simulink model "CompletoyLPV"  (R2025a)
settings: Solver=VariableStepAuto  StartTime=0.0  StopTime=10.0  RelTol=1e-3
PostLoadFcn:
  | parametros_sistema_completo
  | run("parametros_sistema_completo.mlx")
values from neighbouring files (symbols this model uses):
  a_cu = 3.9e-3    (= 0.0039)    [parametros_sistema_completo.m]    (also in workspace_params.mat)
  b_eq = params.b_total    [calcular_matriz_AO.m]    (also in calculo_incertidumbre_y_control.m = b_m + b_l/(r^2); parametros_sistema_completo.m = 2.19444444444e-05; workspace_params.mat = 2.19444444444e-05)
  C_ts = C_ts * (1 + tol_pct)    [calculo_incertidumbre_y_control.m]    (also in parametros_sistema_completo.m = 0.818; workspace_params.mat = 0.818)
  g = 9.80665    [parametros_sistema_completo.m]    (also in workspace_params.mat)
  J_eq = params.J_total    [calcular_matriz_AO.m]    (also in calculo_incertidumbre_y_control.m = J_m + J_l/r^2; parametros_sistema_completo.m = 1.97847222222e-05; workspace_params.mat = 3.28055555556e-05)
  k_l = m*l_cm + m_l*l_l    [calculo_incertidumbre_y_control.m]    (also in parametros_sistema_completo.m = 0.25; workspace_params.mat = 0.625)
  L_d = L_d    * (1 - tol_pct)    [calculo_incertidumbre_y_control.m]    (also in parametros_sistema_completo.m = 0.0066; workspace_params.mat = 0.0066)
  L_ls = L_ls   * (1 - tol_pct)    [calculo_incertidumbre_y_control.m]    (also in parametros_sistema_completo.m = 0.0008; workspace_params.mat = 0.0008)
  L_q = L_q    * (1 - tol_pct)    [calculo_incertidumbre_y_control.m]    (also in parametros_sistema_completo.m = 0.0058; workspace_params.mat = 0.0058)
  lambda_r = lambda_r * (1 + tol_pct)    [calculo_incertidumbre_y_control.m]    (also in parametros_sistema_completo.m = 0.016; workspace_params.mat = 0.016)
  P_p = 3    [parametros_sistema_completo.m]    (also in workspace_params.mat)
  r = params.r_red    [calcular_matriz_AO.m]    (also in parametros_sistema_completo.m = 120; workspace_params.mat = 120)
  R_sREF = R_sREF * (1 - tol_pct)    [calculo_incertidumbre_y_control.m]    (also in parametros_sistema_completo.m = 1.02; workspace_params.mat = 1.02)
  R_ts_amb = R_ts_amb * (1 - tol_pct)    [calculo_incertidumbre_y_control.m]    (also in parametros_sistema_completo.m = 146.7; workspace_params.mat = 146.7)
  s = max(diff(xl),diff(yl)); xlim(mean(xl)+[-1 1]*s/2); ylim(mean(yl)+[-1 1]*s/2); axis square    [mapa_polos_5_2_2.m]    (also in metricas_5_1_6b.m = iqs(idx); modulador_torque_521.m = tf('s'))
  T_amb = 20    [parametros_sistema_completo.m]    (also in workspace_params.mat)
  T_sREF = 20    [parametros_sistema_completo.m]    (also in workspace_params.mat)
undefined symbols (not defined in the file or in its folder): deg, rad
libraries: aerolibconvert2 x1
settings Model: Creator=Francisco  LastModifiedBy=Francisco
settings DebuggingCC: UnderspecifiedInitializationDetection=Classic  MergeDetectMultiDrivingBlocksExec=none
settings ModelReferenceCC: PropagateSignalLabelsOutOfModel=off
settings RTWCC: GPUComputeCapability=3.5

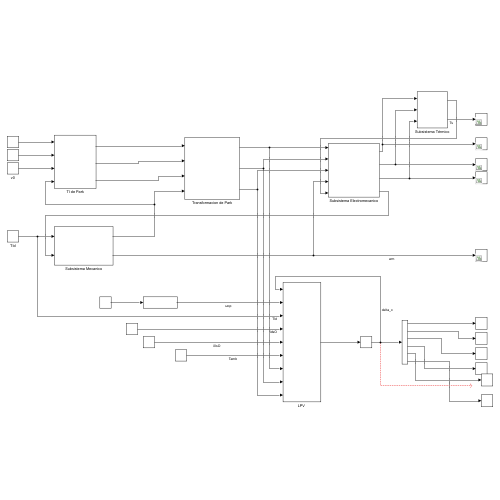
[thumbnail: Simulink's stored preview of the top-level diagram]
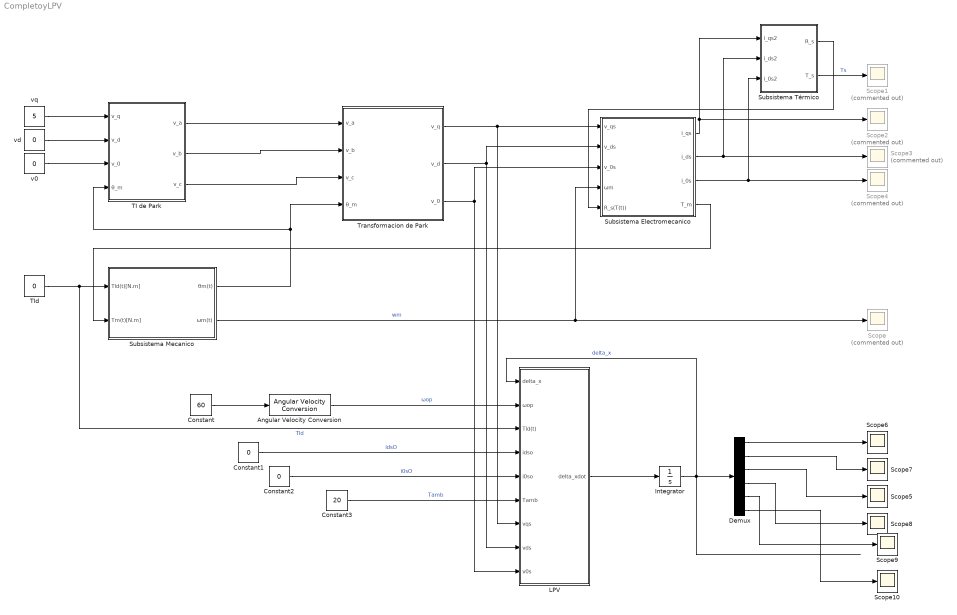
== system CompletoyLPV ==
  Angular Velocity Conversion : aerolibconvert2/Angular Velocity Conversion  IU=deg/s  OU=rad/s
  Constant : Constant  Value=60
  Constant1 : Constant  Value=0
  Constant2 : Constant  Value=0
  Constant3 : Constant  Value=20
  Demux : Demux  Outputs=6
  Integrator : Integrator
  "LPV " : Subsystem
  Scope{,1..4} (5 alike) : Scope  Commented=on
      Scope settings: ActiveDisplayYMinimum=73.83566  ActiveDisplayYMaximum=91.14361
      Scope1 settings: ActiveDisplayYMinimum=-0.21459  ActiveDisplayYMaximum=1.93128
      Scope2 settings: ActiveDisplayYMinimum=-0.79232  ActiveDisplayYMaximum=3.09165  DataLoggingVariableName=ScopeData2
      Scope3 settings: ActiveDisplayYMinimum=-0.21509  ActiveDisplayYMaximum=1.75287  DataLoggingVariableName=ScopeData3
      Scope4 settings: ActiveDisplayYMinimum=-4.8E-11  ActiveDisplayYMaximum=5E-11  DataLoggingVariableName=ScopeData4
  Scope{5..10} (6 alike) : Scope
      Scope10 settings: ActiveDisplayYMinimum=1.2614013021411665  ActiveDisplayYMaximum=31.468208023043097  DataLoggingVariableName=ScopeData10
      Scope5 settings: ActiveDisplayYMinimum=-67.200227328003422  ActiveDisplayYMaximum=44.635452648293487  DataLoggingVariableName=ScopeData5
      Scope6 settings: ActiveDisplayYMinimum=-60.0071453689453  ActiveDisplayYMaximum=12.244259941879115  DataLoggingVariableName=ScopeData6
      Scope7 settings: ActiveDisplayYMinimum=-3.8566133388452828  ActiveDisplayYMaximum=11.094644624657567  DataLoggingVariableName=ScopeData7
      Scope8 settings: ActiveDisplayYMinimum=-4.8085485964497172  ActiveDisplayYMaximum=10.142709367053149  DataLoggingVariableName=ScopeData8
      Scope9 settings: ActiveDisplayYMinimum=-7.1222346828694452  ActiveDisplayYMaximum=12.913880935880563  DataLoggingVariableName=ScopeData9
  Subsistema Electromecanico : Subsystem
  Subsistema Mecanico : Subsystem
  Subsistema Térmico : Subsystem
  TI de Park : Subsystem
  TId : Constant  Value=0
  Transformacion de Park : Subsystem
  v0 : Constant  Value=0
  vd : Constant  Value=0
  vq : Constant  Value=5
  wires:
  Transformacion de Park/3(v_0) -> Subsistema Electromecanico/3(v_0s), "LPV "/9(v0s)
  Transformacion de Park/2(v_d) -> Subsistema Electromecanico/2(v_ds), "LPV "/8(vds)
  Transformacion de Park/1(v_q) -> "LPV "/7(vqs), Subsistema Electromecanico/1(v_qs)
  Subsistema Térmico/1(R_s) -> Subsistema Electromecanico/5(R_s(T(t)))
  Subsistema Electromecanico/2(i_ds) -> Subsistema Térmico/2(i_ds2), Scope3/1
  Subsistema Térmico/2(T_s) -> Scope1/1  "Ts"
  vq/1 -> TI de Park/1(v_q)
  vd/1 -> TI de Park/2(v_d)
  v0/1 -> TI de Park/3(v_0)
  Subsistema Mecanico/1(θm(t)) -> Transformacion de Park/4(θ_m), TI de Park/4(θ_m)
  Subsistema Mecanico/2(ωm(t)) -> Scope/1, Subsistema Electromecanico/4(ωm)  "wm"
  TI de Park/3(v_c) -> Transformacion de Park/3(v_c)
  Subsistema Electromecanico/1(i_qs) -> Scope2/1, Subsistema Térmico/1(i_qs2)
  Subsistema Electromecanico/3(i_0s) -> Scope4/1, Subsistema Térmico/3(i_0s2)
  Subsistema Electromecanico/4(T_m) -> Subsistema Mecanico/2(Tm(t)[N.m])
  TI de Park/1(v_a) -> Transformacion de Park/1(v_a)
  TI de Park/2(v_b) -> Transformacion de Park/2(v_b)
  Angular Velocity Conversion/1 -> "LPV "/2(ωop)  "ωop"
  TId/1 -> "LPV "/3(Tld(t)), Subsistema Mecanico/1(Tld(t)[N.m])  "Tld"
  Constant1/1 -> "LPV "/4(idso)  "idsO"
  Constant2/1 -> "LPV "/5(i0so)  "i0sO"
  Constant3/1 -> "LPV "/6(Tamb)  "Tamb"
  "LPV "/1(delta_xdot) -> Integrator/1
  Integrator/1 -> "LPV "/1(delta_x), Demux/1  "delta_x"
  Constant/1 -> Angular Velocity Conversion/1
  Demux/3 -> Scope5/1
  Demux/1 -> Scope6/1
  Demux/2 -> Scope7/1
  Demux/4 -> Scope8/1
  Demux/5 -> Scope9/1
  Demux/6 -> Scope10/1

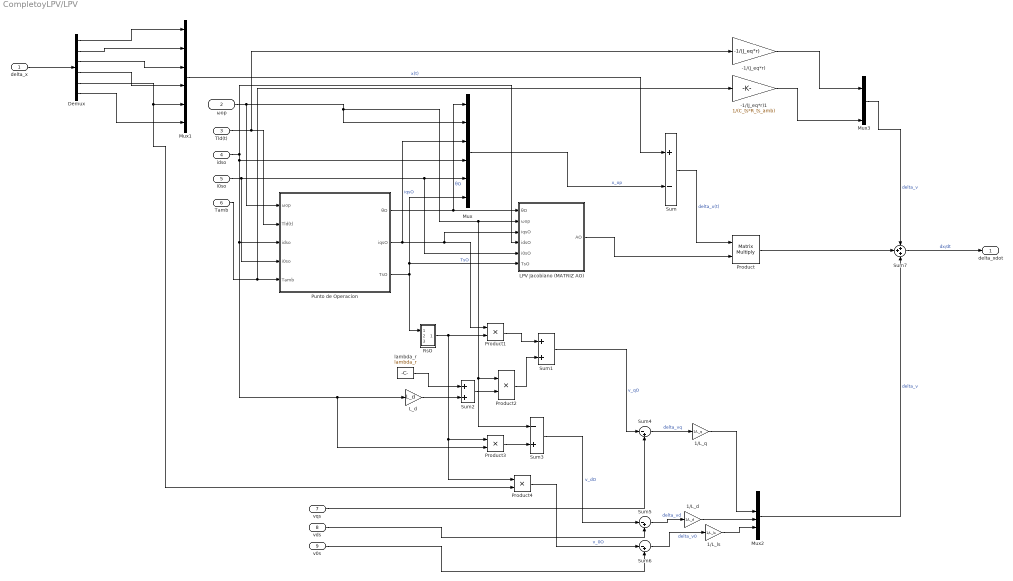
== system CompletoyLPV/LPV  ==
  delta_x : Inport
  ωop : Inport  Port=2
  Tld(t) : Inport  Port=3
  idso : Inport  Port=4
  i0so : Inport  Port=5
  Tamb : Inport  Port=6
  vqs : Inport  Port=7
  vds : Inport  Port=8
  v0s : Inport  Port=9
  -1/(J_eq*r) : Gain  Gain=-1/(J_eq*r)
  -1/(J_eq*r)1 : Gain  Gain=1/(C_ts*R_ts_amb)
  1/L_d : Gain  Gain=1/L_d
  1/L_ls : Gain  Gain=1/L_ls
  1/L_q : Gain  Gain=1/L_q
  Demux : Demux  Outputs=6
  LPV Jacobiano (MATRIZ AO) : Subsystem
  L_d : Gain  Gain=L_d
  Mux{,1..3} (4 alike) : Mux  Inputs=6
  Product : Product  Multiplication=Matrix(*)
  Product{1..4} (4 alike) : Product
  Punto de Operacion : Subsystem
  RsO : MATLAB Function  TreatAsAtomicUnit=on
  Sum : Sum  Inputs=+-
  Sum1 : Sum
  Sum2 : Sum
  Sum3 : Sum  Inputs=-+
  Sum4 : Sum  Inputs=|-+
  Sum5 : Sum  Inputs=|-+
  Sum6 : Sum  Inputs=|-+
  Sum7 : Sum  Inputs=+++
  lambda_r : Constant  Value=lambda_r
  delta_xdot : Outport
  wires:
  Punto de Operacion/2(iqsO) -> Product1/1, LPV Jacobiano (MATRIZ AO)/3(iqsO), Mux/3  "iqsO"
  Mux1/1 -> Sum/1  "x(t)"
  ωop/1 -> Punto de Operacion/1(ωop), LPV Jacobiano (MATRIZ AO)/2(ωop), Sum3/1, Product2/1, Mux/2
  Punto de Operacion/1(θO) -> LPV Jacobiano (MATRIZ AO)/1(θO), Mux/1  "θO"
  Tamb/1 -> -1/(J_eq*r)1/1, Punto de Operacion/5(Tamb)
  i0so/1 -> Mux/5, LPV Jacobiano (MATRIZ AO)/5(i0sO), Punto de Operacion/4(i0so)
  Product/1 -> Sum7/2
  idso/1 -> Mux/4, Punto de Operacion/3(idso), Product3/2, L_d/1, LPV Jacobiano (MATRIZ AO)/4(idsO)
  Mux/1 -> Sum/2  "x_op"
  LPV Jacobiano (MATRIZ AO)/1(AO) -> Product/2
  Sum/1 -> Product/1  "delta_x(t)"
  Tld(t)/1 -> -1/(J_eq*r)/1, Punto de Operacion/2(Tld(t))
  Punto de Operacion/3(TsO) -> RsO/1(TsO), LPV Jacobiano (MATRIZ AO)/6(TsO), Mux/6  "TsO"
  Demux/2 -> Mux1/2
  Demux/6 -> Mux1/6
  Demux/1 -> Mux1/1
  Demux/5 -> Product4/2, Mux1/5
  Demux/4 -> Mux1/4
  Demux/3 -> Mux1/3
  RsO/1(RsO) -> Product4/1, Product3/1, Product1/2
  Product1/1 -> Sum1/1
  L_d/1 -> Sum2/2
  lambda_r/1 -> Sum2/1
  Sum2/1 -> Product2/2
  Product2/1 -> Sum1/2
  Sum1/1 -> Sum4/1  "v_qO"
  Product3/1 -> Sum3/2
  Sum3/1 -> Sum5/1  "v_dO"
  Product4/1 -> Sum6/1  "v_0O"
  vqs/1 -> Sum4/2
  vds/1 -> Sum5/2
  v0s/1 -> Sum6/2
  Mux2/1 -> Sum7/3  "delta_v"
  Sum4/1 -> 1/L_q/1  "delta_vq"
  Sum5/1 -> 1/L_d/1  "delta_vd"
  Sum6/1 -> 1/L_ls/1  "delta_v0"
  1/L_ls/1 -> Mux2/5
  1/L_d/1 -> Mux2/4
  1/L_q/1 -> Mux2/3
  -1/(J_eq*r)/1 -> Mux3/2
  -1/(J_eq*r)1/1 -> Mux3/6
  Mux3/1 -> Sum7/1  "delta_v"
  Sum7/1 -> delta_xdot/1  "dx/dt"
  delta_x/1 -> Demux/1

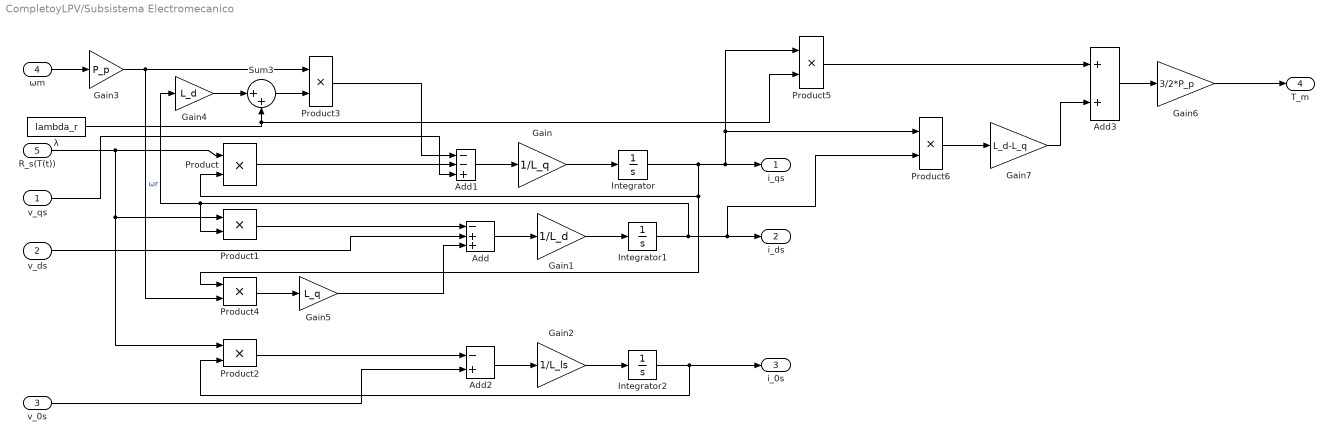
== system CompletoyLPV/Subsistema Electromecanico ==
  v_qs : Inport
  v_ds : Inport  Port=2
  v_0s : Inport  Port=3
  ωm : Inport  Port=4
  R_s(T(t)) : Inport  Port=5
  Add : Sum  Inputs=-++
  Add1 : Sum  Inputs=--+
  Add2 : Sum  Inputs=-+
  Add3 : Sum
  Gain : Gain  Gain=1/L_q
  Gain1 : Gain  Gain=1/L_d
  Gain2 : Gain  Gain=1/L_ls
  Gain3 : Gain  Gain=P_p
  Gain4 : Gain  Gain=L_d
  Gain5 : Gain  Gain=L_q
  Gain6 : Gain  Gain=3/2*P_p
  Gain7 : Gain  Gain=L_d-L_q
  Integrator : Integrator
  Integrator1 : Integrator
  Integrator2 : Integrator
  Product{,1..6} (7 alike) : Product
  Sum3 : Sum  Inputs=|++
  λ : Constant  Value=lambda_r
  i_qs : Outport
  i_ds : Outport  Port=2
  i_0s : Outport  Port=3
  T_m : Outport  Port=4
  wires:
  v_0s/1 -> Add2/2
  Gain5/1 -> Add/3
  Gain3/1 -> Product4/2, Product3/1  "ωr"
  Integrator/1 -> Product4/1, Product/2, i_qs/1, Product5/1, Product6/1
  v_qs/1 -> Add1/3
  R_s(T(t))/1 -> Product2/1, Product1/1, Product/1
  Gain4/1 -> Sum3/1
  Product1/1 -> Add/1
  Integrator2/1 -> i_0s/1, Product2/2
  Sum3/1 -> Product3/2
  Integrator1/1 -> Gain4/1, Product1/2, i_ds/1, Product6/2
  Product/1 -> Add1/2
  Product4/1 -> Gain5/1
  ωm/1 -> Gain3/1
  Add3/1 -> Gain6/1
  Gain/1 -> Integrator/1
  Gain6/1 -> T_m/1
  Product2/1 -> Add2/1
  λ/1 -> Sum3/2, Product5/2
  Gain1/1 -> Integrator1/1
  Add/1 -> Gain1/1
  Add1/1 -> Gain/1
  Product6/1 -> Gain7/1
  Product3/1 -> Add1/1
  Gain2/1 -> Integrator2/1
  Gain7/1 -> Add3/2
  v_ds/1 -> Add/2
  Add2/1 -> Gain2/1
  Product5/1 -> Add3/1

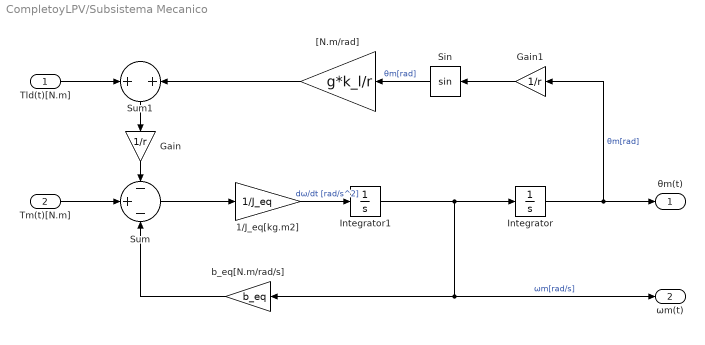
== system CompletoyLPV/Subsistema Mecanico ==
  Tld(t)[N.m] : Inport
  Tm(t)[N.m] : Inport  Port=2
  1/J_eq[kg.m2] : Gain  Gain=1/J_eq
  Gain : Gain  Gain=1/r
  Gain1 : Gain  Gain=1/r
  Integrator : Integrator
  Integrator1 : Integrator
  Sin : Trigonometry
  Sum : Sum  Inputs=-+-
  Sum1 : Sum
  "[N.m/rad]" : Gain  Gain=g*k_l/r
  b_eq[N.m/rad/s] : Gain  Gain=b_eq
  θm(t) : Outport
  ωm(t) : Outport  Port=2
  wires:
  Gain1/1 -> Sin/1
  Sin/1 -> "[N.m/rad]"/1  "θm[rad]"
  Integrator1/1 -> Integrator/1, ωm(t)/1, b_eq[N.m/rad/s]/1  "ωm[rad/s]"
  Tld(t)[N.m]/1 -> Sum1/1
  b_eq[N.m/rad/s]/1 -> Sum/3
  1/J_eq[kg.m2]/1 -> Integrator1/1  "dω/dt [rad/s^2]"
  Gain/1 -> Sum/1
  "[N.m/rad]"/1 -> Sum1/2
  Integrator/1 -> θm(t)/1, Gain1/1  "θm[rad]"
  Sum/1 -> 1/J_eq[kg.m2]/1
  Tm(t)[N.m]/1 -> Sum/2
  Sum1/1 -> Gain/1

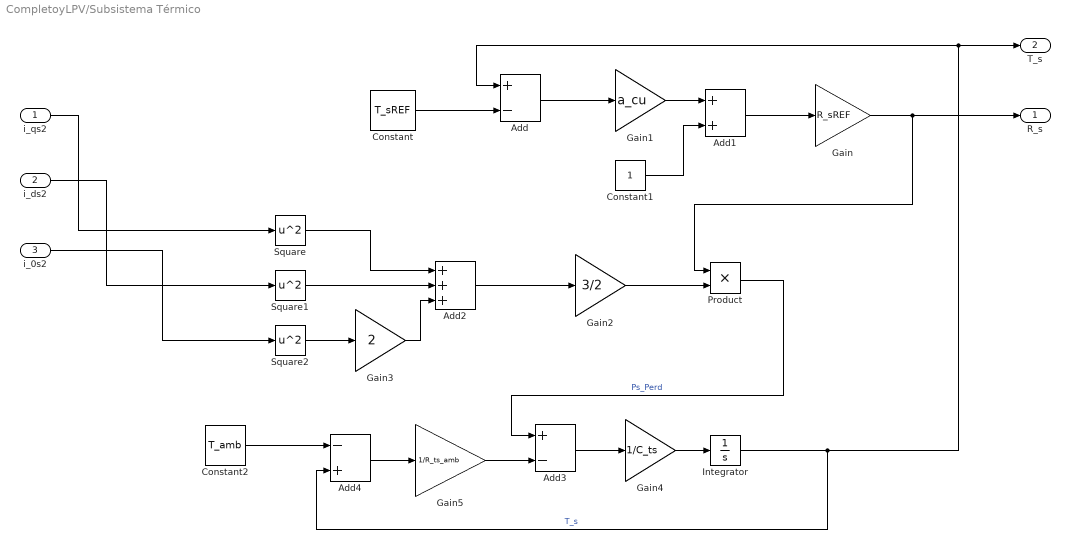
== system CompletoyLPV/Subsistema Térmico ==
  i_qs2 : Inport
  i_ds2 : Inport  Port=2
  i_0s2 : Inport  Port=3
  Add : Sum  Inputs=+-
  Add1 : Sum
  Add2 : Sum  Inputs=+++
  Add3 : Sum  Inputs=+-
  Add4 : Sum  Inputs=-+
  Constant : Constant  Value=T_sREF
  Constant1 : Constant
  Constant2 : Constant  Value=T_amb
  Gain : Gain  Gain=R_sREF
  Gain1 : Gain  Gain=a_cu
  Gain2 : Gain  Gain=3/2
  Gain3 : Gain  Gain=2
  Gain4 : Gain  Gain=1/C_ts
  Gain5 : Gain  Gain=1/R_ts_amb
  Integrator : Integrator
  Product : Product
  Square : Math  Operator=square  OutDataTypeStr=double
  Square1 : Math  Operator=square
  Square2 : Math  Operator=square
  R_s : Outport
  T_s : Outport  Port=2
  wires:
  Constant1/1 -> Add1/2
  Constant/1 -> Add/2
  i_qs2/1 -> Square/1
  Gain/1 -> R_s/1, Product/1
  Square/1 -> Add2/1
  Add2/1 -> Gain2/1
  Constant2/1 -> Add4/1
  i_ds2/1 -> Square1/1
  Gain5/1 -> Add3/2
  Integrator/1 -> Add4/2, T_s/1, Add/1  "T_s"
  Add1/1 -> Gain/1
  i_0s2/1 -> Square2/1
  Square1/1 -> Add2/2
  Product/1 -> Add3/1  "Ps_Perd"
  Gain2/1 -> Product/2
  Add/1 -> Gain1/1
  Square2/1 -> Gain3/1
  Gain1/1 -> Add1/1
  Add3/1 -> Gain4/1
  Add4/1 -> Gain5/1
  Gain3/1 -> Add2/3
  Gain4/1 -> Integrator/1

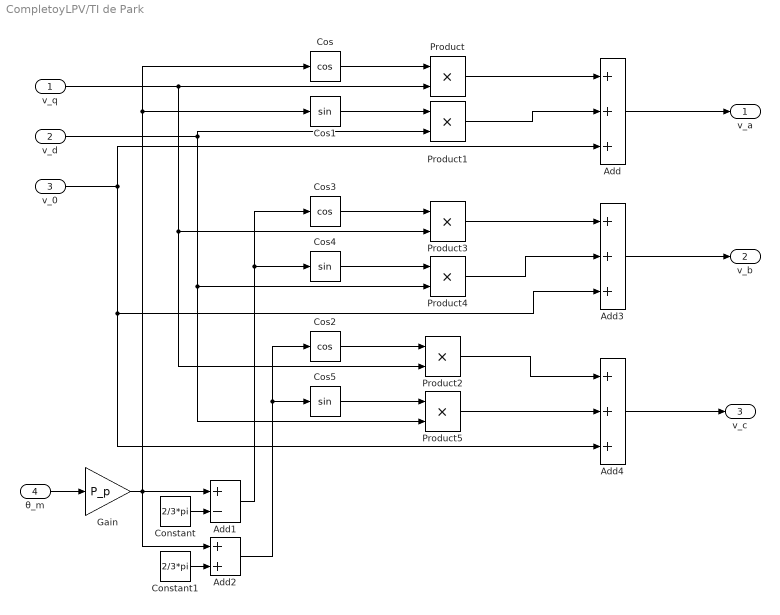
== system CompletoyLPV/TI de Park ==
  v_q : Inport
  v_d : Inport  Port=2
  v_0 : Inport  Port=3
  θ_m : Inport  Port=4
  Add : Sum  Inputs=+++
  Add1 : Sum  Inputs=+-
  Add2 : Sum
  Add3 : Sum  Inputs=+++
  Add4 : Sum  Inputs=+++
  Constant : Constant  Value=2/3*pi
  Constant1 : Constant  Value=2/3*pi
  Cos : Trigonometry  Operator=cos
  Cos1 : Trigonometry
  Cos2 : Trigonometry  Operator=cos
  Cos3 : Trigonometry  Operator=cos
  Cos4 : Trigonometry
  Cos5 : Trigonometry
  Gain : Gain  Gain=P_p
  Product{,1..5} (6 alike) : Product
  v_a : Outport
  v_b : Outport  Port=2
  v_c : Outport  Port=3
  wires:
  Product4/1 -> Add3/2
  Cos1/1 -> Product1/1
  Cos/1 -> Product/1
  Product1/1 -> Add/2
  Add3/1 -> v_b/1
  Cos3/1 -> Product3/1
  Product3/1 -> Add3/1
  v_d/1 -> Product1/2, Product5/2, Product4/2
  Constant1/1 -> Add2/2
  Constant/1 -> Add1/2
  v_0/1 -> Add3/3, Add4/3, Add/3
  Add1/1 -> Cos3/1, Cos4/1
  Product/1 -> Add/1
  v_q/1 -> Product/2, Product2/2, Product3/2
  Cos4/1 -> Product4/1
  Gain/1 -> Add2/1, Add1/1, Cos/1, Cos1/1
  θ_m/1 -> Gain/1
  Add/1 -> v_a/1
  Add4/1 -> v_c/1
  Cos2/1 -> Product2/1
  Cos5/1 -> Product5/1
  Add2/1 -> Cos5/1, Cos2/1
  Product2/1 -> Add4/1
  Product5/1 -> Add4/2

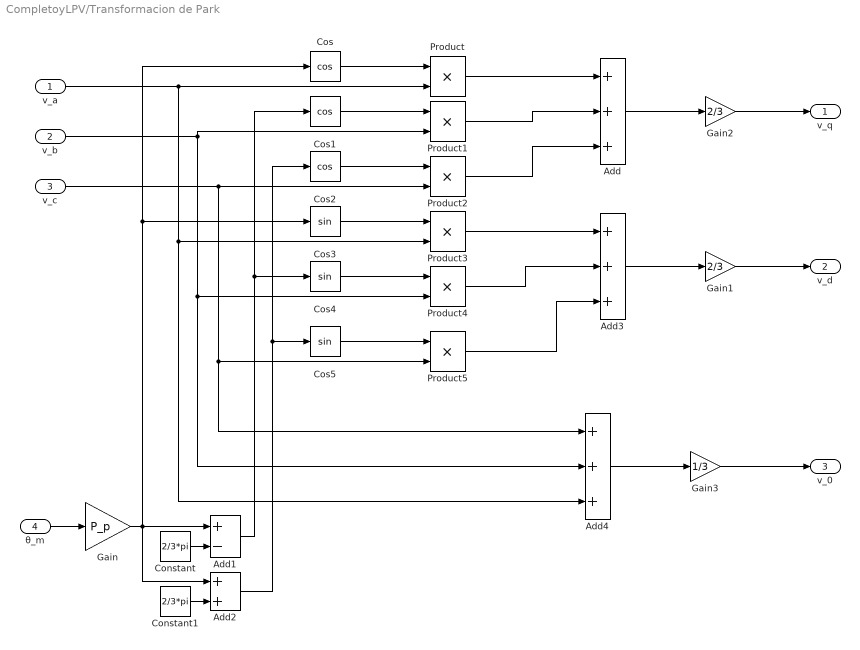
== system CompletoyLPV/Transformacion de Park ==
  v_a : Inport
  v_b : Inport  Port=2
  v_c : Inport  Port=3
  θ_m : Inport  Port=4
  Add : Sum  Inputs=+++
  Add1 : Sum  Inputs=+-
  Add2 : Sum
  Add3 : Sum  Inputs=+++
  Add4 : Sum  Inputs=+++
  Constant : Constant  Value=2/3*pi
  Constant1 : Constant  Value=2/3*pi
  Cos : Trigonometry  Operator=cos
  Cos1 : Trigonometry  Operator=cos
  Cos2 : Trigonometry  Operator=cos
  Cos3 : Trigonometry
  Cos4 : Trigonometry
  Cos5 : Trigonometry
  Gain : Gain  Gain=P_p
  Gain1 : Gain  Gain=2/3
  Gain2 : Gain  Gain=2/3
  Gain3 : Gain  Gain=1/3
  Product{,1..5} (6 alike) : Product
  v_q : Outport
  v_d : Outport  Port=2
  v_0 : Outport  Port=3
  wires:
  θ_m/1 -> Gain/1
  Cos5/1 -> Product5/1
  Gain2/1 -> v_q/1
  Product5/1 -> Add3/3
  Add/1 -> Gain2/1
  Gain/1 -> Cos3/1, Cos/1, Add1/1, Add2/1
  Cos4/1 -> Product4/1
  Cos2/1 -> Product2/1
  v_a/1 -> Add4/3, Product3/2, Product/2
  Product/1 -> Add/1
  Add1/1 -> Cos1/1, Cos4/1
  v_c/1 -> Product2/2, Product5/2, Add4/1
  Constant/1 -> Add1/2
  Constant1/1 -> Add2/2
  v_b/1 -> Product1/2, Product4/2, Add4/2
  Add2/1 -> Cos2/1, Cos5/1
  Add4/1 -> Gain3/1
  Product3/1 -> Add3/1
  Product2/1 -> Add/3
  Gain3/1 -> v_0/1
  Cos3/1 -> Product3/1
  Add3/1 -> Gain1/1
  Gain1/1 -> v_d/1
  Product1/1 -> Add/2
  Cos/1 -> Product/1
  Cos1/1 -> Product1/1
  Product4/1 -> Add3/2

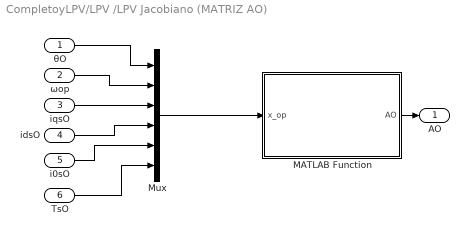
== system CompletoyLPV/LPV /LPV Jacobiano (MATRIZ AO) ==
  θO : Inport
  ωop : Inport  Port=2
  iqsO : Inport  Port=3
  idsO : Inport  Port=4
  i0sO : Inport  Port=5
  TsO : Inport  Port=6
  MATLAB Function : MATLAB Function  TreatAsAtomicUnit=on
  Mux : Mux  Inputs=6
  AO : Outport
  wires:
  Mux/1 -> MATLAB Function/1(x_op)
  MATLAB Function/1(AO) -> AO/1
  idsO/1 -> Mux/4
  iqsO/1 -> Mux/3
  TsO/1 -> Mux/6
  ωop/1 -> Mux/2
  i0sO/1 -> Mux/5
  θO/1 -> Mux/1

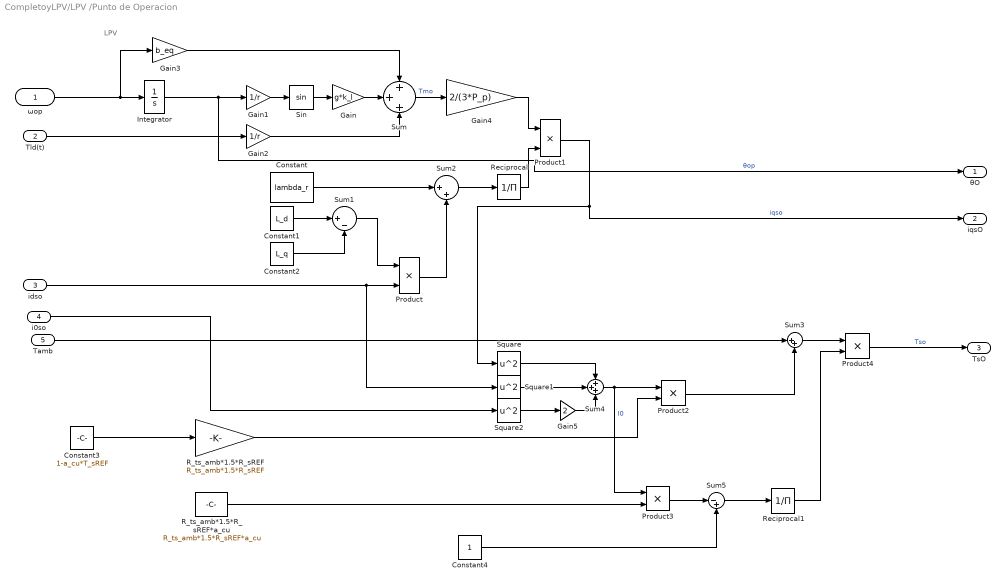
== system CompletoyLPV/LPV /Punto de Operacion ==
  note: LPV
  ωop : Inport
  Tld(t) : Inport  Port=2
  idso : Inport  Port=3
  i0so : Inport  Port=4
  Tamb : Inport  Port=5
  Constant : Constant  Value=lambda_r
  Constant1 : Constant  Value=L_d
  Constant2 : Constant  Value=L_q
  Constant3 : Constant  Value=1-a_cu*T_sREF
  Constant4 : Constant
  Gain : Gain  Gain=g*k_l
  Gain1 : Gain  Gain=1/r
  Gain2 : Gain  Gain=1/r
  Gain3 : Gain  Gain=b_eq
  Gain4 : Gain  Gain=2/(3*P_p)
  Gain5 : Gain  Gain=2
  Integrator : Integrator
  Product{,1..4} (5 alike) : Product
  R_ts_amb*1.5*R_sREF : Gain  Gain=R_ts_amb*1.5*R_sREF
  R_ts_amb*1.5*R_sREF*a_cu : Constant  Value=R_ts_amb*1.5*R_sREF*a_cu
  Reciprocal : Product  Inputs=/
  Reciprocal1 : Product  Inputs=/
  Sin : Trigonometry
  Square : Math  Operator=square
  Square1 : Math  Operator=square
  Square2 : Math  Operator=square
  Sum : Sum  Inputs=+++
  Sum1 : Sum  Inputs=|+-
  Sum2 : Sum  Inputs=|++
  Sum3 : Sum  Inputs=|++
  Sum4 : Sum  Inputs=+++
  Sum5 : Sum  Inputs=|-+
  θO : Outport
  iqsO : Outport  Port=2
  TsO : Outport  Port=3
  wires:
  Constant2/1 -> Sum1/2
  Constant3/1 -> R_ts_amb*1.5*R_sREF/1
  Integrator/1 -> θO/1, Gain1/1  "θop"
  Product1/1 -> iqsO/1, Square/1  "iqso"
  ωop/1 -> Integrator/1, Gain3/1
  Square2/1 -> Gain5/1
  Constant4/1 -> Sum5/2
  Gain5/1 -> Sum4/3
  Sum1/1 -> Product/1
  Sum3/1 -> Product4/1
  Gain3/1 -> Sum/1
  Sin/1 -> Gain/1
  idso/1 -> Product/2, Square1/1
  Reciprocal/1 -> Product1/2
  Product4/1 -> TsO/1  "Tso"
  Square/1 -> Sum4/1
  Gain/1 -> Sum/2
  Product/1 -> Sum2/2
  Square1/1 -> Sum4/2
  Sum/1 -> Gain4/1  "Tmo"
  Gain1/1 -> Sin/1
  Constant/1 -> Sum2/1
  Constant1/1 -> Sum1/1
  Sum4/1 -> Product3/1, Product2/1  "I0"
  Tamb/1 -> Sum3/1
  Tld(t)/1 -> Gain2/1
  Sum2/1 -> Reciprocal/1
  Sum5/1 -> Reciprocal1/1
  Gain2/1 -> Sum/3
  Product3/1 -> Sum5/1
  Gain4/1 -> Product1/1
  R_ts_amb*1.5*R_sREF/1 -> Product2/2
  R_ts_amb*1.5*R_sREF*a_cu/1 -> Product3/2
  i0so/1 -> Square2/1
  Product2/1 -> Sum3/2
  Reciprocal1/1 -> Product4/2

== matlab function CompletoyLPV/LPV /RsO ==
  data: TsO input; RsO output; a_cu input; T_sREF input; R_sREF parameter
function RsO = RsO(TsO,a_cu,T_sREF, R_sREF)
RsO = R_sREF*(1+a_cu*(TsO-T_sREF));

== matlab function CompletoyLPV/LPV /LPV Jacobiano (MATRIZ AO)/MATLAB Function ==
  data: x_op input; AO output; params parameter
function AO = calcular_matriz_AO(x_op, params)
    % Entradas:
    % x_op: Vector del punto de operación [theta_mO; w_mO; i_qsO; i_dsO; i_0sO; TsO]
    % params: Estructura con constantes (Ld, Lq, Rs_ref, etc.)
    
    % 1. Desempaquetar el Punto de Operación (Operating Point)
    theta_mO = x_op(1);
    w_mO     = x_op(2);
    i_qsO    = x_op(3);
    i_dsO    = x_op(4);
    i_0sO    = x_op(5);
    % Nota: TsO (Temperatura) suele ser una entrada exógena o estado lento.
    % Si la linealización incluye la dinámica térmica, se usa x_op(6).
    % Si no, TsO es un parámetro que varía lento. Asumimos estado x_op(6) 
    % por tu matriz de 6x6.
    TsO      = x_op(6); 

    % 2. Desempaquetar parámetros (o usar params.Variable)
    Ld      = params.Ld;
    Lq      = params.Lq;
    Lls     = params.Lls;
    Rs_ref  = params.Rs_ref;
    alpha_cu= params.alpha_cu;
    lambda_m= params.lambda_m;
    Pp      = params.Pp;
    J_eq    = params.J_total; % Inercia total
    b_eq    = params.b_total; % Fricción total
    r       = params.r_red;
    kl      = params.kl;      % Constante de carga (m*g*l_cm...)
    g       = params.g;
    Cts     = params.Cts;
    Rts_amb = params.Rts_amb;
    
    % 3. Cálculo auxiliar de Rs en el punto de operación
    % (Necesario para los términos que no son derivadas parciales de R)
    % Ec. [cite_start]3.9 de la guía [cite: 103]
    % Asumiendo T_ref = 20 grados (o el valor que tengas en params)
    delta_T = TsO - params.Ts_ref;
    Rs_op   = Rs_ref * (1 + alpha_cu * delta_T);

    % 4. Cálculo de Gamma_th (Elemento A(6,6))
    % Definición dada en tu ecuación
    term_currents = 2*(i_0sO^2) + i_dsO^2 + i_qsO^2;
    Gamma_th = -((1/Rts_amb) - (3/2)*Rs_ref*alpha_cu*term_currents) / Cts;

    % 5. Construcción de la Matriz AO (6x6)
    % Inicializamos en ceros para eficiencia
    AO = zeros(6,6);

    % Fila 1: Derivada de Theta (Velocidad)
    AO(1,2) = 1;

    % Fila 2: Derivada de Omega (Mecánica)
    % Termino d(Tm)/d(theta) (Gravedad linealizada)
    AO(2,1) = -(g * kl * cos(theta_mO / r)) / (J_eq * r^2); 
    % Fricción viscosa
    AO(2,2) = -b_eq / J_eq;
    % Acoplamiento corriente q (Torque)
    AO(2,3) = (1.5 * Pp * (lambda_m + i_dsO*(Ld - Lq))) / J_eq;
    % Acoplamiento corriente d (Torque de reluctancia)
    AO(2,4) = (1.5 * Pp * i_qsO * (Ld - Lq)) / J_eq;

    % Fila 3: Derivada de i_qs (Eje q)
    % Acoplamiento w (f.c.e.m.)
    AO(3,2) = -(Pp * (lambda_m + Ld * i_dsO)) / Lq;
    % Resistencia / Inductancia
    AO(3,3) = -Rs_op / Lq;
    % Acoplamiento eje d
    AO(3,4) = -(Ld * Pp * w_mO) / Lq;
    % Sensibilidad térmica de R
    AO(3,6) = -(Rs_ref * alpha_cu * i_qsO) / Lq;

    % Fila 4: Derivada de i_ds (Eje d)
    % Acoplamiento eje q
    AO(4,2) = (Lq * Pp * i_qsO) / Ld; % OJO: En tu imagen dice Lq*Pp*i_qs0 / Ld en pos(4,2)?
    % Nota: Revisa si este termino depende de w o de i_qs. 
    % La derivada de (w*Lq*iq) respecto a w es Lq*iq. Correcto.
    
    AO(4,3) = (Lq * Pp * w_mO) / Ld;
    AO(4,4) = -Rs_op / Ld;
    AO(4,6) = -(Rs_ref * alpha_cu * i_dsO) / Ld;

    % Fila 5: Derivada de i_0s (Secuencia cero)
    % Si el neutro flota, i_0s suele ser 0 y desacoplada, pero incluimos tu ec.
    AO(5,5) = -Rs_op / Lls;
    AO(5,6) = -(Rs_ref * alpha_cu * i_0sO) / Lls;

    % Fila 6: Derivada de Temperatura
    % Joule losses derivatives
    AO(6,3) = (3 * Rs_op * i_qsO) / Cts;
    AO(6,4) = (3 * Rs_op * i_dsO) / Cts;
    AO(6,5) = (6 * Rs_op * i_0sO) / Cts; % Factor 6 según tu fórmula (3 fases * 2?)
    AO(6,6) = Gamma_th;

end
